simulink model "roll_sim"  (R2013a)
settings: Solver=ode45  StartTime=0.0  StopTime=2  RelTol=1e-3
values from neighbouring files (symbols this model uses):
  b = 0.002    [PSAS_Rocket_sys.m]    (also in lqrQfinder.m = 0.02; roll_sys.m; rotational_system.m = 0.02; stevens_state_space_for_rocket.m = [J^-1*Tb])
  fr = 2.75*.0254    (= 0.06985)    [PSAS_Rocket_sys.m]    (also in lqrQfinder.m; roll_sys.m; rotational_system.m = 0.0635)
  Ftot = 7    [roll_sys.m]    (also in rotational_system.m = 5.5)
  hz = 5    [PSAS_Rocket_sys.m]    (also in roll_sys.m; rotational_system.m = 10)
  I = 1/2*m*r^2    (= 0.0197946818182)    [lqrQfinder.m]    (also in roll_sys.m = 0.0198; rotational_system.m = 0.075)
  Tau = 0.02    [roll_sys.m]    (also in rotational_system.m = 0.009)
libraries: simulink x2
settings Model: Creator=karnell  LastModifiedBy=kenny
settings DataIOCC: SignalLoggingSaveFormat=ModelDataLogs
settings DebuggingCC: MultiTaskDSMMsg=warning  MultiTaskCondExecSysMsg=none  StateNameClashWarn=none  StrictBusMsg=None
settings RTWCC: IncludeERTFirstTime=on

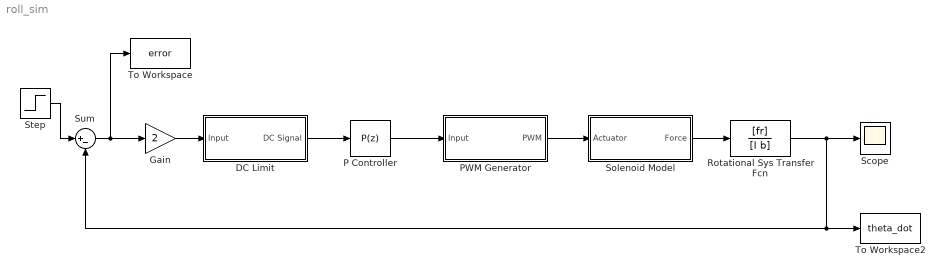
== system roll_sim ==
  DC Limit : Subsystem
  Gain : Gain  Gain=2
  P Controller : simulink/Continuous/PID Controller  Controller=P  TimeDomain=Discrete-time  SampleTime=.003  IntegratorMethod=Forward Euler  FilterMethod=Forward Euler  Form=Parallel  P=.2  I=0  D=0  N=100  InitialConditionSource=internal  InitialConditionForIntegrator=0  InitialConditionForFilter=0  ExternalReset=none  LimitOutput=off  UpperSaturationLimit=inf  LowerSaturationLimit=-inf  LinearizeAsGain=on  AntiWindupMode=none  Kb=1  TrackingMode=off  Kt=1  PParamMin=[]  PParamMax=[]  IParamMin=[]  IParamMax=[]  DParamMin=[]  DParamMax=[]  NParamMin=[]  NParamMax=[]  KbParamMin=[]  KbParamMax=[]  KtParamMin=[]  KtParamMax=[]  POutMin=[]  POutMax=[]  IOutMin=[]  IOutMax=[]  DOutMin=[]  DOutMax=[]  NOutMin=[]  NOutMax=[]  KbOutMin=[]  KbOutMax=[]  KtOutMin=[]  KtOutMax=[]  IntegratorOutMin=[]  IntegratorOutMax=[]  FilterOutMin=[]  FilterOutMax=[]  SumOutMin=[]  SumOutMax=[]  SumI1OutMin=[]  SumI1OutMax=[]  SumI2OutMin=[]  SumI2OutMax=[]  SumI3OutMin=[]  SumI3OutMax=[]  SumDOutMin=[]  SumDOutMax=[]  SaturationOutMin=[]  SaturationOutMax=[]  IntegratorContinuousStateAttributes=''  IntegratorStateMustResolveToSignalObject=off  IntegratorRTWStateStorageClass=Auto  FilterContinuousStateAttributes=''  FilterStateMustResolveToSignalObject=off  FilterRTWStateStorageClass=Auto
  PWM Generator : Subsystem
  Rotational Sys Transfer Fcn : TransferFcn  Numerator=[fr]  Denominator=[I b]
  Scope : Scope
      settings: SaveName=ScopeData3
  Solenoid Model : Subsystem
  Step : Step  Time=0  After=1.03  SampleTime=0
  Sum : Sum  Inputs=|+-
  To Workspace : ToWorkspace  VariableName=error  SampleTime=-1  SaveFormat=Structure With Time
  To Workspace2 : ToWorkspace  VariableName=theta_dot  SampleTime=-1  SaveFormat=Structure With Time
  wires:
  Sum/1 -> Gain/1, To Workspace/1
  PWM Generator/1(PWM) -> Solenoid Model/1(Actuator)
  DC Limit/1(DC Signal) -> P Controller/1
  Step/1 -> Sum/1
  Rotational Sys Transfer Fcn/1 -> Scope/1, To Workspace2/1, Sum/2
  P Controller/1 -> PWM Generator/1(Input)
  Gain/1 -> DC Limit/1(Input)
  Solenoid Model/1(Force) -> Rotational Sys Transfer Fcn/1

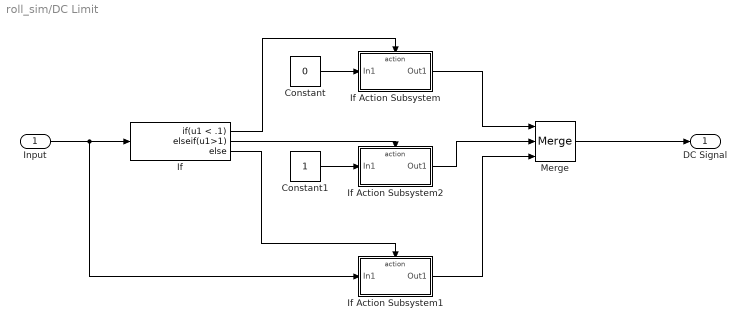
== system roll_sim/DC Limit ==
  Input : Inport
  Constant : Constant  Value=0
  Constant1 : Constant
  If : If  IfExpression=u1 < .1  ElseIfExpressions=u1>1
  If Action Subsystem : Subsystem  TreatAsAtomicUnit=on
  If Action Subsystem1 : Subsystem  TreatAsAtomicUnit=on
  If Action Subsystem2 : Subsystem  TreatAsAtomicUnit=on
  Merge : Merge  Inputs=3
  DC Signal : Outport
  wires:
  Input/1 -> If Action Subsystem1/1(In1), If/1
  Merge/1 -> DC Signal/1
  If Action Subsystem/1(Out1) -> Merge/1
  Constant/1 -> If Action Subsystem/1(In1)
  If/1 -> If Action Subsystem/Action
  If/3 -> If Action Subsystem1/Action
  If Action Subsystem1/1(Out1) -> Merge/3
  If/2 -> If Action Subsystem2/Action
  If Action Subsystem2/1(Out1) -> Merge/2
  Constant1/1 -> If Action Subsystem2/1(In1)

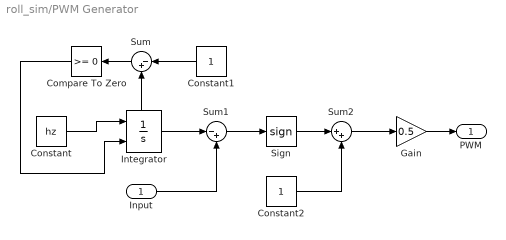
== system roll_sim/PWM Generator ==
  Input : Inport
  Compare To Zero : simulink/Logic and Bit Operations/Compare To Zero  relop=>=  OutDataTypeStr=boolean
  Constant : Constant  Value=hz
  Constant1 : Constant
  Constant2 : Constant
  Gain : Gain  Gain=0.5
  Integrator : Integrator  ExternalReset=rising  ShowStatePort=on
  Sign : Signum
  Sum : Sum  Inputs=|-+
  Sum1 : Sum  Inputs=|-+
  Sum2 : Sum  Inputs=|++
  PWM : Outport
  wires:
  Constant1/1 -> Sum/1
  Sum/1 -> Compare To Zero/1
  Integrator/1 -> Sum1/1
  Input/1 -> Sum1/2
  Sum1/1 -> Sign/1
  Sign/1 -> Sum2/1
  Constant2/1 -> Sum2/2
  Sum2/1 -> Gain/1
  Gain/1 -> PWM/1
  Constant/1 -> Integrator/1
  Compare To Zero/1 -> Integrator/2
  Integrator/State -> Sum/2

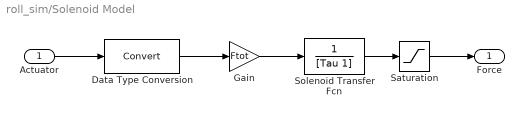
== system roll_sim/Solenoid Model ==
  Actuator : Inport
  Data Type Conversion : DataTypeConversion
  Gain : Gain  Gain=Ftot
  Saturation : Saturate  UpperLimit=Ftot  LowerLimit=-Ftot
  Solenoid Transfer Fcn : TransferFcn  Denominator=[Tau 1]
  Force : Outport
  wires:
  Gain/1 -> Solenoid Transfer Fcn/1
  Saturation/1 -> Force/1
  Data Type Conversion/1 -> Gain/1
  Solenoid Transfer Fcn/1 -> Saturation/1
  Actuator/1 -> Data Type Conversion/1

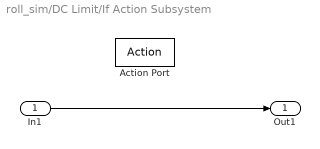
== system roll_sim/DC Limit/If Action Subsystem ==
  In1 : Inport
  Action Port : ActionPort  ActionType=then
  Out1 : Outport
  wires:
  In1/1 -> Out1/1

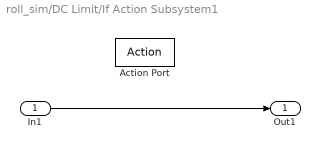
== system roll_sim/DC Limit/If Action Subsystem1 ==
  In1 : Inport
  Action Port : ActionPort  ActionType=else
  Out1 : Outport
  wires:
  In1/1 -> Out1/1

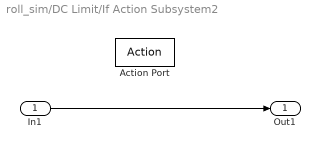
== system roll_sim/DC Limit/If Action Subsystem2 ==
  In1 : Inport
  Action Port : ActionPort  ActionType=elseif
  Out1 : Outport
  wires:
  In1/1 -> Out1/1
